simulink subsystem "rss_PwrTubPCBTempHiLvl2Dia"  (R2023a)
settings: Solver=VariableStepAuto  StartTime=0.0  StopTime=10.0  RelTol=1e-3
undefined symbols (not defined in the file): ENM_TYPE_FALT, Gu16_ctPCBTempHiLvl2ConfCnt_C, Gu16_ctPCBTempHiLvl2RcvyCnt_C, Gu16_ctPwrTubTempHiLvl2ConfCnt_C, Gu16_ctPwrTubTempHiLvl2RcvyCnt_C, Gu8_tPCBTempHiLvl2ConfTrs_C, Gu8_tPCBTempHiLvl2RcvyTrs_C, Gu8_tPwrTubTempHiLvl2ConfTrs_C, Gu8_tPwrTubTempHiLvl2RcvyTrs_C
libraries: vhit_control_library x2, lib_fault_definiteness x2
settings Model: Creator=xiaoqiang.yuan  LastModifiedBy=xiaoqiang.yuan

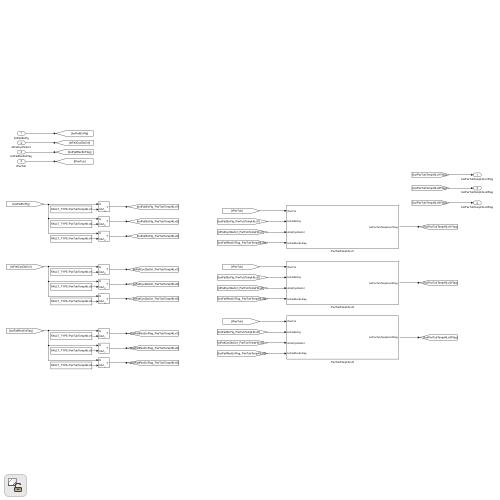
[thumbnail: Simulink's stored preview of the top-level diagram]
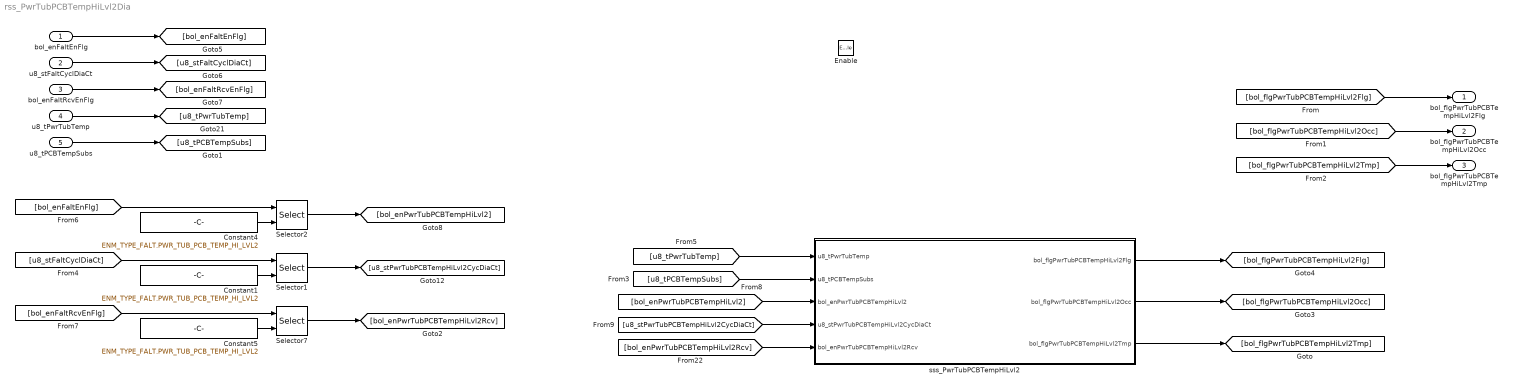
== system rss_PwrTubPCBTempHiLvl2Dia ==
  bol_enFaltEnFlg : Inport  OutDataTypeStr=boolean
  u8_stFaltCyclDiaCt : Inport  Port=2  OutDataTypeStr=uint8
  bol_enFaltRcvEnFlg : Inport  Port=3  OutDataTypeStr=boolean
  u8_tPwrTubTemp : Inport  Port=4  OutDataTypeStr=dt_Temp_u8p0bn40
  u8_tPCBTempSubs : Inport  Port=5  OutDataTypeStr=dt_Temp_u8p0bn40
  Enable : EnablePort
  Constant1 : Constant  Value=ENM_TYPE_FALT.PWR_TUB_PCB_TEMP_HI_LVL2
  Constant4 : Constant  Value=ENM_TYPE_FALT.PWR_TUB_PCB_TEMP_HI_LVL2
  Constant5 : Constant  Value=ENM_TYPE_FALT.PWR_TUB_PCB_TEMP_HI_LVL2
  Selector1 : Selector  IndexMode=Zero-based  InputPortWidth=Cdbl_numFaltDiaNum  IndexOptions=Index vector (port)  Indices=[1 3]  OutputSizes=1
  Selector2 : Selector  IndexMode=Zero-based  InputPortWidth=Cdbl_numFaltDiaNum  IndexOptions=Index vector (port)  Indices=[1 3]  OutputSizes=1
  Selector7 : Selector  IndexMode=Zero-based  InputPortWidth=Cdbl_numFaltDiaNum  IndexOptions=Index vector (port)  Indices=[1 3]  OutputSizes=1
  sss_PwrTubPCBTempHiLvl2 : Subsystem
  bol_flgPwrTubPCBTempHiLvl2Flg : Outport  OutDataTypeStr=boolean
  bol_flgPwrTubPCBTempHiLvl2Occ : Outport  Port=2  OutDataTypeStr=boolean
  bol_flgPwrTubPCBTempHiLvl2Tmp : Outport  Port=3  OutDataTypeStr=boolean
  wires:
  [bol_flgPwrTubPCBTempHiLvl2Flg] -> bol_flgPwrTubPCBTempHiLvl2Flg/1
  u8_tPwrTubTemp/1 -> [u8_tPwrTubTemp]
  Selector2/1 -> [bol_enPwrTubPCBTempHiLvl2]
  [bol_enFaltEnFlg] -> Selector2/1
  [bol_enPwrTubPCBTempHiLvl2] -> sss_PwrTubPCBTempHiLvl2/3(bol_enPwrTubPCBTempHiLvl2)
  Constant4/1 -> Selector2/2
  [u8_stPwrTubPCBTempHiLvl2CycDiaCt] -> sss_PwrTubPCBTempHiLvl2/4(u8_stPwrTubPCBTempHiLvl2CycDiaCt)
  [u8_tPwrTubTemp] -> sss_PwrTubPCBTempHiLvl2/1(u8_tPwrTubTemp)
  bol_enFaltEnFlg/1 -> [bol_enFaltEnFlg]
  bol_enFaltRcvEnFlg/1 -> [bol_enFaltRcvEnFlg]
  u8_stFaltCyclDiaCt/1 -> [u8_stFaltCyclDiaCt]
  [bol_enPwrTubPCBTempHiLvl2Rcv] -> sss_PwrTubPCBTempHiLvl2/5(bol_enPwrTubPCBTempHiLvl2Rcv)
  Selector1/1 -> [u8_stPwrTubPCBTempHiLvl2CycDiaCt]
  Constant1/1 -> Selector1/2
  [u8_stFaltCyclDiaCt] -> Selector1/1
  Selector7/1 -> [bol_enPwrTubPCBTempHiLvl2Rcv]
  Constant5/1 -> Selector7/2
  [bol_enFaltRcvEnFlg] -> Selector7/1
  sss_PwrTubPCBTempHiLvl2/1(bol_flgPwrTubPCBTempHiLvl2Flg) -> [bol_flgPwrTubPCBTempHiLvl2Flg]
  u8_tPCBTempSubs/1 -> [u8_tPCBTempSubs]
  [u8_tPCBTempSubs] -> sss_PwrTubPCBTempHiLvl2/2(u8_tPCBTempSubs)
  sss_PwrTubPCBTempHiLvl2/2(bol_flgPwrTubPCBTempHiLvl2Occ) -> [bol_flgPwrTubPCBTempHiLvl2Occ]
  [bol_flgPwrTubPCBTempHiLvl2Occ] -> bol_flgPwrTubPCBTempHiLvl2Occ/1
  [bol_flgPwrTubPCBTempHiLvl2Tmp] -> bol_flgPwrTubPCBTempHiLvl2Tmp/1
  sss_PwrTubPCBTempHiLvl2/3(bol_flgPwrTubPCBTempHiLvl2Tmp) -> [bol_flgPwrTubPCBTempHiLvl2Tmp]

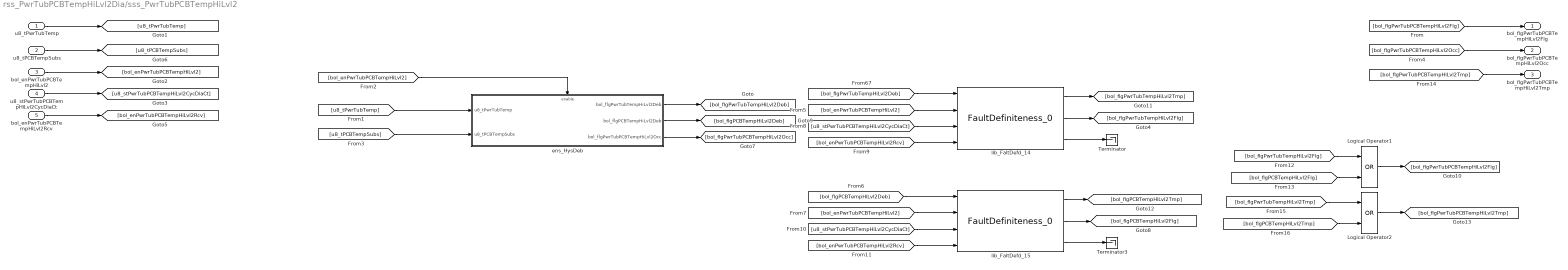
== system rss_PwrTubPCBTempHiLvl2Dia/sss_PwrTubPCBTempHiLvl2 ==
  u8_tPwrTubTemp : Inport
  u8_tPCBTempSubs : Inport  Port=2
  bol_enPwrTubPCBTempHiLvl2 : Inport  Port=3
  u8_stPwrTubPCBTempHiLvl2CycDiaCt : Inport  Port=4
  bol_enPwrTubPCBTempHiLvl2Rcv : Inport  Port=5
  Logical Operator1 : Logic  Operator=OR  AllPortsSameDT=off  OutDataTypeStr=boolean
  Logical Operator2 : Logic  Operator=OR  AllPortsSameDT=off  OutDataTypeStr=boolean
  Terminator : Terminator
  Terminator3 : Terminator
  ens_HysDeb : Subsystem
  lib_FaltDefd_14 : lib_fault_definiteness/FaultDefiniteness_0  lb_FaltWaitRecvCnt=Gu16_ctPwrTubTempHiLvl2ConfCnt_C
  lib_FaltDefd_15 : lib_fault_definiteness/FaultDefiniteness_0  lb_FaltWaitRecvCnt=Gu16_ctPCBTempHiLvl2ConfCnt_C
  bol_flgPwrTubPCBTempHiLvl2Flg : Outport
  bol_flgPwrTubPCBTempHiLvl2Occ : Outport  Port=2
  bol_flgPwrTubPCBTempHiLvl2Tmp : Outport  Port=3  OutDataTypeStr=boolean
  wires:
  Logical Operator2/1 -> [bol_flgPwrTubPCBTempHiLvl2Tmp]
  [bol_flgPCBTempHiLvl2Tmp] -> Logical Operator2/2
  [bol_flgPwrTubTempHiLvl2Tmp] -> Logical Operator2/1
  [bol_flgPwrTubPCBTempHiLvl2Tmp] -> bol_flgPwrTubPCBTempHiLvl2Tmp/1
  Logical Operator1/1 -> [bol_flgPwrTubPCBTempHiLvl2Flg]
  [bol_flgPCBTempHiLvl2Flg] -> Logical Operator1/2
  [bol_flgPwrTubTempHiLvl2Flg] -> Logical Operator1/1
  [bol_enPwrTubPCBTempHiLvl2Rcv] -> lib_FaltDefd_15/4
  [u8_stPwrTubPCBTempHiLvl2CycDiaCt] -> lib_FaltDefd_15/3
  [bol_enPwrTubPCBTempHiLvl2] -> lib_FaltDefd_15/2
  lib_FaltDefd_15/3 -> Terminator3/1
  lib_FaltDefd_15/1 -> [bol_flgPCBTempHiLvl2Tmp]
  lib_FaltDefd_15/2 -> [bol_flgPCBTempHiLvl2Flg]
  [bol_flgPCBTempHiLvl2Deb] -> lib_FaltDefd_15/1
  ens_HysDeb/2(bol_flgPCBTempHiLvl2Deb) -> [bol_flgPCBTempHiLvl2Deb]
  [bol_flgPwrTubPCBTempHiLvl2Occ] -> bol_flgPwrTubPCBTempHiLvl2Occ/1
  ens_HysDeb/3(bol_flgPwrTubPCBTempHiLvl2Occ) -> [bol_flgPwrTubPCBTempHiLvl2Occ]
  [u8_tPCBTempSubs] -> ens_HysDeb/2(u8_tPCBTempSubs)
  u8_tPCBTempSubs/1 -> [u8_tPCBTempSubs]
  lib_FaltDefd_14/1 -> [bol_flgPwrTubTempHiLvl2Tmp]
  lib_FaltDefd_14/2 -> [bol_flgPwrTubTempHiLvl2Flg]
  lib_FaltDefd_14/3 -> Terminator/1
  [bol_enPwrTubPCBTempHiLvl2] -> ens_HysDeb/Enable
  [u8_tPwrTubTemp] -> ens_HysDeb/1(u8_tPwrTubTemp)
  ens_HysDeb/1(bol_flgPwrTubTempHiLvl2Deb) -> [bol_flgPwrTubTempHiLvl2Deb]
  bol_enPwrTubPCBTempHiLvl2Rcv/1 -> [bol_enPwrTubPCBTempHiLvl2Rcv]
  u8_stPwrTubPCBTempHiLvl2CycDiaCt/1 -> [u8_stPwrTubPCBTempHiLvl2CycDiaCt]
  bol_enPwrTubPCBTempHiLvl2/1 -> [bol_enPwrTubPCBTempHiLvl2]
  [bol_flgPwrTubPCBTempHiLvl2Flg] -> bol_flgPwrTubPCBTempHiLvl2Flg/1
  u8_tPwrTubTemp/1 -> [u8_tPwrTubTemp]
  [bol_enPwrTubPCBTempHiLvl2Rcv] -> lib_FaltDefd_14/4
  [u8_stPwrTubPCBTempHiLvl2CycDiaCt] -> lib_FaltDefd_14/3
  [bol_enPwrTubPCBTempHiLvl2] -> lib_FaltDefd_14/2
  [bol_flgPwrTubTempHiLvl2Deb] -> lib_FaltDefd_14/1

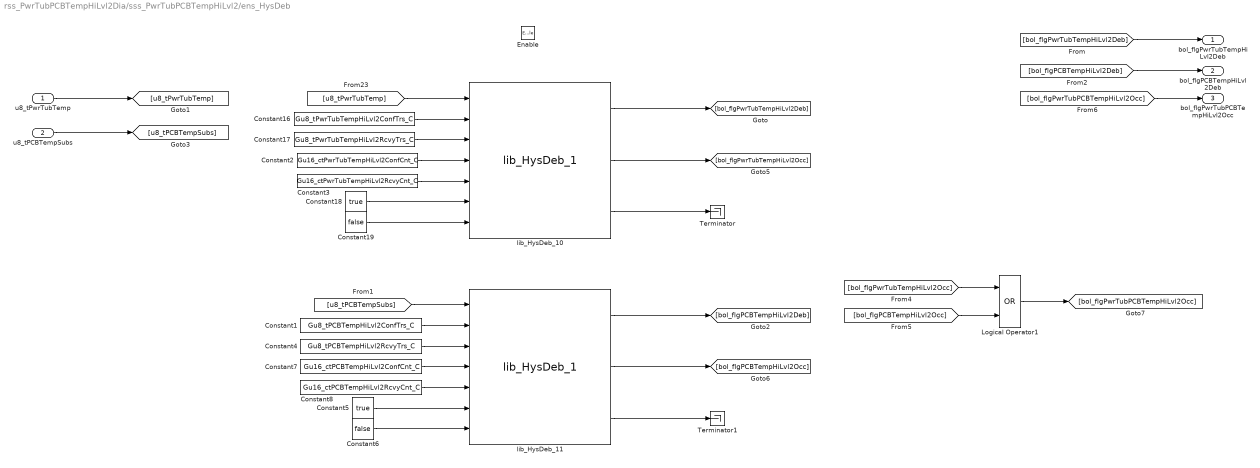
== system rss_PwrTubPCBTempHiLvl2Dia/sss_PwrTubPCBTempHiLvl2/ens_HysDeb ==
  u8_tPwrTubTemp : Inport
  u8_tPCBTempSubs : Inport  Port=2
  Enable : EnablePort
  Constant1 : Constant  Value=Gu8_tPCBTempHiLvl2ConfTrs_C
  Constant16 : Constant  Value=Gu8_tPwrTubTempHiLvl2ConfTrs_C
  Constant17 : Constant  Value=Gu8_tPwrTubTempHiLvl2RcvyTrs_C
  Constant18 : Constant  Value=true  OutDataTypeStr=boolean
  Constant19 : Constant  Value=false  OutDataTypeStr=boolean
  Constant2 : Constant  Value=Gu16_ctPwrTubTempHiLvl2ConfCnt_C
  Constant3 : Constant  Value=Gu16_ctPwrTubTempHiLvl2RcvyCnt_C
  Constant4 : Constant  Value=Gu8_tPCBTempHiLvl2RcvyTrs_C
  Constant5 : Constant  Value=true  OutDataTypeStr=boolean
  Constant6 : Constant  Value=false  OutDataTypeStr=boolean
  Constant7 : Constant  Value=Gu16_ctPCBTempHiLvl2ConfCnt_C
  Constant8 : Constant  Value=Gu16_ctPCBTempHiLvl2RcvyCnt_C
  Logical Operator1 : Logic  Operator=OR  AllPortsSameDT=off  OutDataTypeStr=boolean
  Terminator : Terminator
  Terminator1 : Terminator
  lib_HysDeb_10 : vhit_control_library/lib_HysDeb_1  lb_parInitOutp=0
  lib_HysDeb_11 : vhit_control_library/lib_HysDeb_1  lb_parInitOutp=0
  bol_flgPwrTubTempHiLvl2Deb : Outport
  bol_flgPCBTempHiLvl2Deb : Outport  Port=2
  bol_flgPwrTubPCBTempHiLvl2Occ : Outport  Port=3
  wires:
  [bol_flgPCBTempHiLvl2Deb] -> bol_flgPCBTempHiLvl2Deb/1
  [bol_flgPwrTubPCBTempHiLvl2Occ] -> bol_flgPwrTubPCBTempHiLvl2Occ/1
  Logical Operator1/1 -> [bol_flgPwrTubPCBTempHiLvl2Occ]
  [bol_flgPCBTempHiLvl2Occ] -> Logical Operator1/2
  [bol_flgPwrTubTempHiLvl2Occ] -> Logical Operator1/1
  lib_HysDeb_11/2 -> [bol_flgPCBTempHiLvl2Occ]
  lib_HysDeb_11/3 -> Terminator1/1
  lib_HysDeb_10/2 -> [bol_flgPwrTubTempHiLvl2Occ]
  lib_HysDeb_10/1 -> [bol_flgPwrTubTempHiLvl2Deb]
  lib_HysDeb_10/3 -> Terminator/1
  [u8_tPCBTempSubs] -> lib_HysDeb_11/1
  Constant7/1 -> lib_HysDeb_11/4
  Constant1/1 -> lib_HysDeb_11/2
  lib_HysDeb_11/1 -> [bol_flgPCBTempHiLvl2Deb]
  u8_tPCBTempSubs/1 -> [u8_tPCBTempSubs]
  Constant5/1 -> lib_HysDeb_11/6
  Constant6/1 -> lib_HysDeb_11/7
  Constant4/1 -> lib_HysDeb_11/3
  Constant8/1 -> lib_HysDeb_11/5
  Constant3/1 -> lib_HysDeb_10/5
  Constant2/1 -> lib_HysDeb_10/4
  Constant19/1 -> lib_HysDeb_10/7
  Constant18/1 -> lib_HysDeb_10/6
  Constant17/1 -> lib_HysDeb_10/3
  Constant16/1 -> lib_HysDeb_10/2
  [u8_tPwrTubTemp] -> lib_HysDeb_10/1
  u8_tPwrTubTemp/1 -> [u8_tPwrTubTemp]
  [bol_flgPwrTubTempHiLvl2Deb] -> bol_flgPwrTubTempHiLvl2Deb/1
